simulink model "Torque_Control"  (R2022a)
settings: Solver=FixedStepAuto  StartTime=0.0  StopTime=10.0  RelTol=1e-3
libraries: simulink x9, eeGeneralControl x3
(part 2 of 6)

== system Torque_Control/Power Limitation Temperature/temperature_SoP/temperature_rise_limitator_Motors ==
  note: initial_limitation es una constante para la reducción inicial (de 0 a 1, más bajo significa que cambia
      | menos, más alto la limitación
      | inicial es más bestia).
  note: saturamos de 1 a 0 por si acaso
  note: magia chunga para
      | que los números cuadren
  note: Se limita la corriente en proporción
      | al ratio entre la temperatura actual y 110ºC
  note: output 0 si está por
      | debajo de 110ºC, 1 si está
      | por encima
  max_motor_temp : Inport
  initial_limitation : Inport  Port=2
  Add1 : Sum  Inputs=-+
  Add2 : Sum  Inputs=-++
  Add3 : Sum  Inputs=+-
  Constant1 : Constant  Value=105
  Constant2 : Constant  Value=5
  Constant3 : Constant
  Divide : Product  Inputs=*/
  Low-Pass Filter (Discrete or Continuous) : eeGeneralControl/Low-Pass Filter (Discrete or Continuous)  K=1  T=100  B=inf  A=-inf  init_option=Inherited from block input  x0=0  Ts=-1
  Product4 : Product
  Saturation1 : Saturate  UpperLimit=1  LowerLimit=0
  Temp higher than 110 : simulink/Logic and Bit Operations/Compare To Constant  relop=>=  const=110  OutDataTypeStr=boolean  ZeroCross=off
  SoP : Outport
  wires:
  Divide/1 -> Add3/1
  Constant3/1 -> Add2/3
  Constant1/1 -> Divide/1
  max_motor_temp/1 -> Add1/2, Temp higher than 110/1
  Temp higher than 110/1 -> Add2/1, Product4/2
  Constant2/1 -> Add1/1
  Product4/1 -> Add2/2
  Add2/1 -> Low-Pass Filter (Discrete or Continuous)/1
  Add3/1 -> Product4/1
  Add1/1 -> Divide/2
  Saturation1/1 -> SoP/1
  initial_limitation/1 -> Add3/2
  Low-Pass Filter (Discrete or Continuous)/1 -> Saturation1/1

== system Torque_Control/SAFETY BLOCK/APPS_IMPLAUSIBILITY/Imp ==
  Action Port : ActionPort  ActionPortLabel=if { }
  Constant : Constant  Value=0  OutDataTypeStr=boolean
  Out1 : Outport  VectorParamsAs1DForOutWhenUnconnected=off
  wires:
  Constant/1 -> Out1/1  "Boolean"

== system Torque_Control/SAFETY BLOCK/APPS_IMPLAUSIBILITY/Not Imp ==
  Action Port : ActionPort  ActionPortLabel=else { }
  Constant : Constant  OutDataTypeStr=boolean
  Out1 : Outport  VectorParamsAs1DForOutWhenUnconnected=off
  wires:
  Constant/1 -> Out1/1  "Boolean"

== system Torque_Control/VDC/Regeneration_Enable/Enabled  ==
  In1 : Inport
  Action Port : ActionPort  ActionPortLabel=if { }
  Out1 : Outport  VectorParamsAs1DForOutWhenUnconnected=off
  wires:
  In1/1 -> Out1/1

== system Torque_Control/VDC/Regeneration_Enable/NotEnabled ==
  In1 : Inport
  Action Port : ActionPort  ActionPortLabel=else { }
  Out1 : Outport  VectorParamsAs1DForOutWhenUnconnected=off
  wires:
  In1/1 -> Out1/1

== system Torque_Control/VDC/TEST_MODE_IN/BYPASS ==
  In1 : Inport
  In2 : Inport  Port=2
  In3 : Inport  Port=3
  In4 : Inport  Port=4
  Action Port : ActionPort  ActionPortLabel=else { }
  Out1 : Outport  VectorParamsAs1DForOutWhenUnconnected=off
  Out2 : Outport  Port=2  VectorParamsAs1DForOutWhenUnconnected=off
  Out3 : Outport  Port=3  VectorParamsAs1DForOutWhenUnconnected=off
  Out4 : Outport  Port=4  VectorParamsAs1DForOutWhenUnconnected=off
  wires:
  In1/1 -> Out1/1
  In2/1 -> Out2/1
  In3/1 -> Out3/1
  In4/1 -> Out4/1

== system Torque_Control/VDC/TEST_MODE_IN/TEST_CONSTANTS ==
  Action Port : ActionPort  ActionPortLabel=if { }
  Constant{,1..3} (4 alike) : Constant  Value=800
  Out1 : Outport  VectorParamsAs1DForOutWhenUnconnected=off
  Out2 : Outport  Port=2  VectorParamsAs1DForOutWhenUnconnected=off
  Out3 : Outport  Port=3  VectorParamsAs1DForOutWhenUnconnected=off
  Out4 : Outport  Port=4  VectorParamsAs1DForOutWhenUnconnected=off
  wires:
  Constant/1 -> Out1/1
  Constant1/1 -> Out2/1
  Constant2/1 -> Out3/1
  Constant3/1 -> Out4/1

== system Torque_Control/VDC/Vehicle Dynamics Control Modes/Automatic Failure Mode ==
  In1 : Inport
  Action Port : ActionPort  ActionPortLabel=if { }
  Out1 : Outport  VectorParamsAs1DForOutWhenUnconnected=off
  wires:
  In1/1 -> Out1/1

== system Torque_Control/VDC/Vehicle Dynamics Control Modes/Manual Failure Mode Selection ==
  In1 : Inport
  Action Port : ActionPort  ActionPortLabel=else { }
  Out1 : Outport  VectorParamsAs1DForOutWhenUnconnected=off
  wires:
  In1/1 -> Out1/1

== system Torque_Control/VDC/Vehicle Dynamics Control Modes/Rigid Axle ==
  "Ap_Sat_up " : Inport
  Ap_Sat_down : Inport  Port=2
  Gas Pedal [0-1] : Inport  Port=3
  Max_Motor_Torque_Rear_FM4 [Nm] : Inport  Port=4
  Gear_Ratio_MtoW : Inport  Port=5
  Action Port : ActionPort  ActionPortLabel=elseif { }
  "Rigid Axle without TC " : MATLAB Function  TreatAsAtomicUnit=on
  Tq_RR_FM4 [Nm] (0,inf) : Outport  VectorParamsAs1DForOutWhenUnconnected=off
  Tq_RL_FM4 [Nm] (0,inf) : Outport  Port=2  VectorParamsAs1DForOutWhenUnconnected=off
  wires:
  Max_Motor_Torque_Rear_FM4 [Nm]/1 -> "Rigid Axle without TC "/4(Maximum_Torque_Rear)
  "Rigid Axle without TC "/2(Torque_RL) -> Tq_RL_FM4 [Nm] (0,inf)/1
  "Rigid Axle without TC "/1(Torque_RR) -> Tq_RR_FM4 [Nm] (0,inf)/1
  Gas Pedal [0-1]/1 -> "Rigid Axle without TC "/1(Ap)
  "Ap_Sat_up "/1 -> "Rigid Axle without TC "/2(Ap_Sat_up)
  Ap_Sat_down/1 -> "Rigid Axle without TC "/3(Ap_Sat_down)
  Gear_Ratio_MtoW/1 -> "Rigid Axle without TC "/5(Transmission_Gear_Ratio)

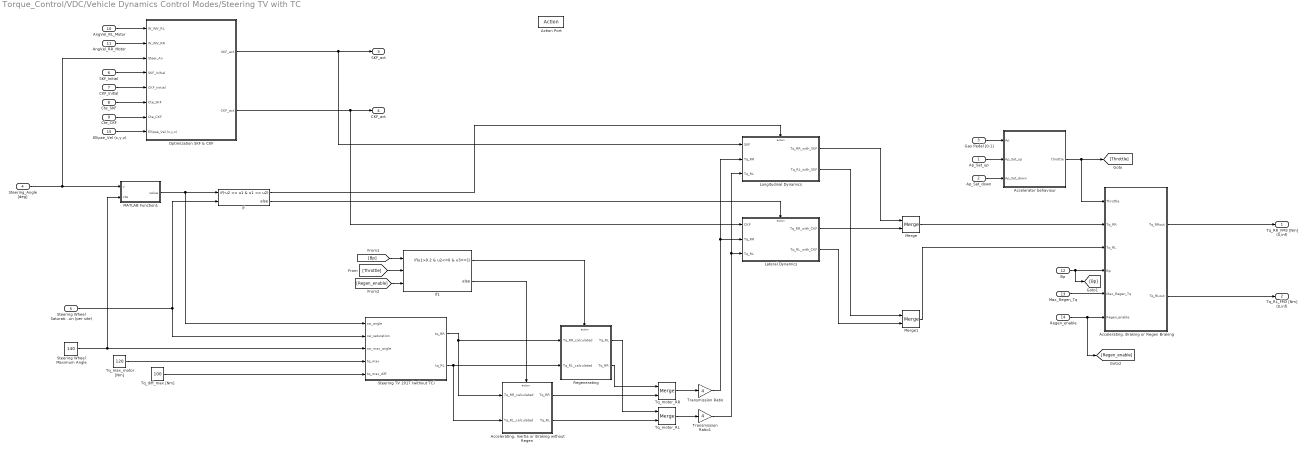
== system Torque_Control/VDC/Vehicle Dynamics Control Modes/Steering TV with TC ==
  "Ap_Sat_up " : Inport
  Ap_Sat_down : Inport  Port=2
  Gas Pedal [0-1] : Inport  Port=3
  Steering_Angle [deg] : Inport  Port=4
  "Steering Wheel Saturation (per site) " : Inport  Port=5
  SKF_Initial : Inport  Port=6
  CKF_Initial : Inport  Port=7
  Cte_SKF : Inport  Port=8
  Cte_CKF : Inport  Port=9
  AngVel_RL_Motor : Inport  Port=10
  AngVel_RR_Motor : Inport  Port=11
  Bp : Inport  Port=12
  Max_Regen_Tq : Inport  Port=13
  Regen_enable : Inport  Port=14
  Ellipse_Vel (x,y,z) : Inport  Port=15
  Action Port : ActionPort  ActionPortLabel=elseif { }
  "Accelerating, Braking or Regen Braking" : Subsystem
  "Accelerating, Inertia or Braking without Regen" : Subsystem  TreatAsAtomicUnit=on
  Accelerator behaviour : MATLAB Function  TreatAsAtomicUnit=on
  If : If  NumInputs=2  IfExpression=-u2 <= u1 & u1 <= u2
  If1 : If  NumInputs=3  IfExpression=u1>0.2 & u2<=0 & u3==1
  Lateral Dynamics : Subsystem  TreatAsAtomicUnit=on
  Longitudinal Dynamics : Subsystem  TreatAsAtomicUnit=on
  MATLAB Function1 : MATLAB Function  TreatAsAtomicUnit=on
  Merge : Merge
  Merge1 : Merge
  Optimization SKF & CKF : Subsystem
  Regenerating : Subsystem  TreatAsAtomicUnit=on
  Steering TV 2017 (without TC) : MATLAB Function  TreatAsAtomicUnit=on
  Steering Wheel Maximum Angle : Constant  Value=140
  Tq_diff_max [Nm] : Constant  Value=100
  Tq_max_motor [Nm] : Constant  Value=120
  Tq_motor_RL : Merge
  Tq_motor_RR : Merge
  Transmission Ratio : Gain  Gain=4
  Transmission Ratio1 : Gain  Gain=4
  Tq_RR_FM3 [Nm] (0,inf) : Outport  VectorParamsAs1DForOutWhenUnconnected=off
  Tq_RL_FM3 [Nm] (0,inf) : Outport  Port=2  VectorParamsAs1DForOutWhenUnconnected=off
  SKF_act : Outport  Port=3  VectorParamsAs1DForOutWhenUnconnected=off
  CKF_act : Outport  Port=4  VectorParamsAs1DForOutWhenUnconnected=off
  wires:
  Steering Wheel Maximum Angle/1 -> Steering TV 2017 (without TC)/3(sw_max_angle), MATLAB Function1/2(cte)
  "Steering Wheel Saturation (per site) "/1 -> Steering TV 2017 (without TC)/2(sw_saturation), If/2
  Transmission Ratio/1 -> Longitudinal Dynamics/2(Tq_RR), Lateral Dynamics/2(Tq_RR)
  Tq_motor_RL/1 -> Transmission Ratio1/1
  MATLAB Function1/1(value) -> Steering TV 2017 (without TC)/1(sw_angle), If/1
  Optimization SKF & CKF/2(CKF_act) -> Lateral Dynamics/1(CKF), CKF_act/1
  SKF_Initial/1 -> Optimization SKF & CKF/4(SKF_Initial)
  Cte_SKF/1 -> Optimization SKF & CKF/6(Cte_SKF)
  AngVel_RL_Motor/1 -> Optimization SKF & CKF/1(W_INV_RL)
  AngVel_RR_Motor/1 -> Optimization SKF & CKF/2(W_INV_RR)
  Optimization SKF & CKF/1(SKF_act) -> Longitudinal Dynamics/1(SKF), SKF_act/1
  Steering_Angle [deg]/1 -> MATLAB Function1/1(v), Optimization SKF & CKF/3(Steer_An)
  CKF_Initial/1 -> Optimization SKF & CKF/5(CKF_Initial)
  Cte_CKF/1 -> Optimization SKF & CKF/7(Cte_CKF)
  If/1 -> Longitudinal Dynamics/Action
  Lateral Dynamics/2(Tq_RL_with_CKF) -> Merge1/2
  If/2 -> Lateral Dynamics/Action
  Longitudinal Dynamics/2(Tq_RL_with_SKF) -> Merge1/1
  Longitudinal Dynamics/1(Tq_RR_with_SKF) -> Merge/1
  Lateral Dynamics/1(Tq_RR_with_CKF) -> Merge/2
  Merge/1 -> "Accelerating, Braking or Regen Braking"/2(Tq_RR)
  Merge1/1 -> "Accelerating, Braking or Regen Braking"/3("Tq_RL ")
  "Accelerating, Braking or Regen Braking"/1(Tq_RRout) -> Tq_RR_FM3 [Nm] (0,inf)/1
  "Accelerating, Braking or Regen Braking"/2(Tq_RLout) -> Tq_RL_FM3 [Nm] (0,inf)/1
  Bp/1 -> [Bp], "Accelerating, Braking or Regen Braking"/4(Bp)
  Max_Regen_Tq/1 -> "Accelerating, Braking or Regen Braking"/5(Max_Regen_Tq)
  Regen_enable/1 -> [Regen_enable], "Accelerating, Braking or Regen Braking"/6(Regen_enable)
  Gas Pedal [0-1]/1 -> Accelerator behaviour/1(Ap)
  "Ap_Sat_up "/1 -> Accelerator behaviour/2(Ap_Sat_up)
  Ap_Sat_down/1 -> Accelerator behaviour/3(Ap_Sat_down)
  Accelerator behaviour/1(throttle) -> [Throttle], "Accelerating, Braking or Regen Braking"/1(Throttle)
  [Throttle] -> If1/2
  [Bp] -> If1/1
  [Regen_enable] -> If1/3
  If1/1 -> Regenerating/Action
  If1/2 -> "Accelerating, Inertia or Braking without Regen"/Action
  Steering TV 2017 (without TC)/2(tq_RL) -> "Accelerating, Inertia or Braking without Regen"/2(Tq_RL_calculated), Regenerating/2(Tq_RL_calculated)
  Steering TV 2017 (without TC)/1(tq_RR) -> "Accelerating, Inertia or Braking without Regen"/1(Tq_RR_calculated), Regenerating/1(Tq_RR_calculated)
  Regenerating/2(Tq_RR) -> Tq_motor_RR/1
  "Accelerating, Inertia or Braking without Regen"/1(Tq_RR) -> Tq_motor_RR/2
  Regenerating/1(Tq_RL) -> Tq_motor_RL/1
  "Accelerating, Inertia or Braking without Regen"/2(Tq_RL) -> Tq_motor_RL/2
  Tq_max_motor [Nm]/1 -> Steering TV 2017 (without TC)/4(tq_max)
  Tq_diff_max [Nm]/1 -> Steering TV 2017 (without TC)/5(tq_max_diff)
  Tq_motor_RR/1 -> Transmission Ratio/1
  Transmission Ratio1/1 -> Longitudinal Dynamics/3(Tq_RL), Lateral Dynamics/3(Tq_RL)
  Ellipse_Vel (x,y,z)/1 -> Optimization SKF & CKF/8(Ellipse_Vel (x,y,z))

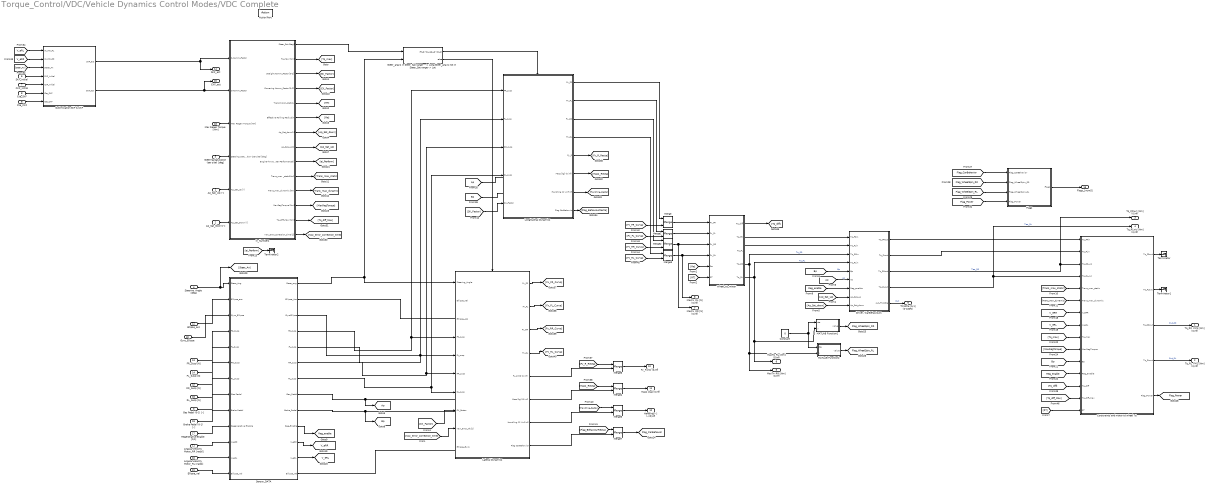
== system Torque_Control/VDC/Vehicle Dynamics Control Modes/VDC Complete ==
  Ap_Sat_Up [-] : Inport
  Ap_Sat_Down [-] : Inport  Port=2
  Gas Pedal (0-1) [-] : Inport  Port=3
  Steering_Angle [deg] : Inport  Port=4
  Steering Saturation (per site) [deg] : Inport  Port=5
  SKF_Initial : Inport  Port=6
  CKF_Initial : Inport  Port=7
  Cte_SKF : Inport  Port=8
  Cte_CKF : Inport  Port=9
  AngularVelocity_Motor_RL [rad/s] : Inport  Port=10
  AngularVelocity_Motor_RR [rad/s] : Inport  Port=11
  Ellipse_acc : Inport  Port=12
  FR_Susp [N] : Inport  Port=13
  FL_Susp [N] : Inport  Port=14
  RR_Susp [N] : Inport  Port=15
  RL_Susp [N] : Inport  Port=16
  Regenerative Enable [0,1] : Inport  Port=17
  Max Regen Torque [Nm] : Inport  Port=18
  Brake Pedal (0-1) [-] : Inport  Port=19
  Gyro_Ellipse : Inport  Port=20
  Ellipse_vel : Inport  Port=21
  Action Port : ActionPort  ActionPortLabel=if { }
  Constant : Constant  Value=0
  Constraints and motor to wheel Tq : Subsystem
  Driver / CarBehaviours : Subsystem
  Flags : Subsystem
  In_Numbers : Subsystem
  Lateral Dynamics : Subsystem  TreatAsAtomicUnit=on
  Longitudinal Dynamics : Subsystem  TreatAsAtomicUnit=on
  MATLAB Function1 : MATLAB Function  TreatAsAtomicUnit=on
  MATLAB Function2 : MATLAB Function  TreatAsAtomicUnit=on
  Merge{,1..7} (8 alike) : Merge
  Optimization SKF & CKF : Subsystem
  Sensor_DATA : Subsystem
  "Steer_ang is in Steer_Sat range ---> Long Steer_ang is not in Steer_Sat range -> Lat " : If  NumInputs=2  IfExpression=u2>=-u1&u2<=u1
  Terminator : Terminator
  Terminator1 : Terminator
  Terminator2 : Terminator
  Wheel_to_motor : Subsystem
  Tq_RR_FM1 [Nm] (0,inf) : Outport  VectorParamsAs1DForOutWhenUnconnected=off
  Tq_RL_FM1 [Nm] (0,inf) : Outport  Port=2  VectorParamsAs1DForOutWhenUnconnected=off
  Tq_RRwc [Nm] (0,inf) : Outport  Port=3  VectorParamsAs1DForOutWhenUnconnected=off
  Tq_RLwc [Nm] (0,inf) : Outport  Port=4  VectorParamsAs1DForOutWhenUnconnected=off
  MaxTq_RR [Nm] (0,inf) : Outport  Port=5  VectorParamsAs1DForOutWhenUnconnected=off
  MaxTq_RL [Nm] (0,inf) : Outport  Port=6  VectorParamsAs1DForOutWhenUnconnected=off
  MaxFx_RR [N] (0,inf) : Outport  Port=7  VectorParamsAs1DForOutWhenUnconnected=off
  MaxFx_RL [N] (0,inf) : Outport  Port=8  VectorParamsAs1DForOutWhenUnconnected=off
  Throttle [0-1] (0-100%) : Outport  Port=9  VectorParamsAs1DForOutWhenUnconnected=off
  Fy_R [N] (0,inf) : Outport  Port=10  VectorParamsAs1DForOutWhenUnconnected=off
  Mass [kg] (0,inf) : Outport  Port=11  VectorParamsAs1DForOutWhenUnconnected=off
  Handling [-] (-inf,inf) : Outport  Port=12  VectorParamsAs1DForOutWhenUnconnected=off
  Flags_[num5] : Outport  Port=13  VectorParamsAs1DForOutWhenUnconnected=off
  SKF_act : Outport  Port=14  VectorParamsAs1DForOutWhenUnconnected=off
  CKF_act : Outport  Port=15  VectorParamsAs1DForOutWhenUnconnected=off
  tag scope: Ap=global, Bp=global, Flag_CarBehavior=global, Flag_Power=global, Flag_WheelSpin_RL=global, Flag_WheelSpin_RR=global, Reg_enable=global, V_eRL=global, V_eRR=global
  wires:
  "Steer_ang is in Steer_Sat range ---> Long Steer_ang is not in Steer_Sat range -> Lat "/1 -> Longitudinal Dynamics/Action
  "Steer_ang is in Steer_Sat range ---> Long Steer_ang is not in Steer_Sat range -> Lat "/2 -> Lateral Dynamics/Action
  Sensor_DATA/7(RL_susp) -> Longitudinal Dynamics/4(RL_susp), Lateral Dynamics/7(RL_susp)
  In_Numbers/3(Straight Kamm_Factor [0-2]) -> [SK_Factor]
  In_Numbers/1(Steer_Sat [deg]) -> "Steer_ang is in Steer_Sat range ---> Long Steer_ang is not in Steer_Sat range -> Lat "/1
  In_Numbers/2(Tq_Max [Nm]) -> [Tq_max]
  Sensor_DATA/8(Gas_Pedal) -> [Ap]
  In_Numbers/6(Effective Rolling Radius[m]) -> [Re]
  In_Numbers/5(Transmision_Ratio[-]) -> [RT]
  Sensor_DATA/6(RR_susp) -> Lateral Dynamics/6(RR_susp), Longitudinal Dynamics/3(RR_susp)
  In_Numbers/8(Ap_Sat_up[-]) -> [Ap_Sat_up]
  In_Numbers/7(Ap_Sat_down[-]) -> [Ap_Sat_down]
  Driver / CarBehaviours/3(Tq_RRout) -> Tq_RRwc [Nm] (0,inf)/1, Constraints and motor to wheel Tq/3(Tq_RR_wc)  "Teo_RR"
  Sensor_DATA/9(Brake_Pedal) -> [Bp]
  Sensor_DATA/5(FL_susp) -> Longitudinal Dynamics/2(FL_susp), Lateral Dynamics/5(FL_susp)
  Sensor_DATA/10(Reg_Enable) -> [Reg_enable]
  Sensor_DATA/4(FR_susp) -> Lateral Dynamics/4(FR_susp), Longitudinal Dynamics/1(FR_susp)
  Sensor_DATA/1(Steer_ang) -> "Steer_ang is in Steer_Sat range ---> Long Steer_ang is not in Steer_Sat range -> Lat "/2, Lateral Dynamics/1(Steering_Angle)
  Wheel_to_motor/5(Tq_RL) -> Driver / CarBehaviours/4("Tq_RLin "), MaxTq_RL [Nm] (0,inf)/1, MATLAB Function1/2(v)  "Tq_RL"
  [Trans_max_dynamic] -> Constraints and motor to wheel Tq/6(Trans_max_dynamic)
  Driver / CarBehaviours/5(out_Throttle) -> Throttle [0-1] (0-100%)/1  "Out"
  Wheel_to_motor/4(Tq_RR) -> Driver / CarBehaviours/3(Tq_RRin), MaxTq_RR [Nm] (0,inf)/1, MATLAB Function2/2(v)  "Tq_RR"
  Wheel_to_motor/3(Tq_FL) -> Driver / CarBehaviours/2(Tq_FLin)
  In_Numbers/11(Trans_max_dynamic [Nm]) -> [Trans_max_dynamic]
  [Reg_enable] -> Driver / CarBehaviours/7(Reg_enable)
  [Ap_Sat_up] -> Driver / CarBehaviours/8(Ap_Sat_up)
  In_Numbers/10(Trans_max _static[Nm]) -> [Trans_max_static]
  [Ap] -> Driver / CarBehaviours/6(Ap)  "Ap"
  [Ap_Sat_down] -> Driver / CarBehaviours/9(Ap_Sat_down)
  Driver / CarBehaviours/4(Tq_RLout) -> Constraints and motor to wheel Tq/4("Tq_RL_wc "), Tq_RLwc [Nm] (0,inf)/1  "Teo_RL"
  Driver / CarBehaviours/2("Tq_FLout ") -> Constraints and motor to wheel Tq/2(Tq_FLin)
  Steering_Angle [deg]/1 -> Sensor_DATA/1(Steer_Ang), [Steer_An]
  Wheel_to_motor/2(Tq_FR) -> Driver / CarBehaviours/1(Tq_FRin)
  Driver / CarBehaviours/1(Tq_FRout) -> Constraints and motor to wheel Tq/1(Tq_FRin)
  [Trans_max_static] -> Constraints and motor to wheel Tq/5("Trans_max_static ")
  [Bp] -> Constraints and motor to wheel Tq/11(Bp)
  Sensor_DATA/12(V_eRL) -> [V_eRL]
  In_Numbers/12(MaxRegTorque [Nm]) -> [MaxRegTorque]
  [Reg_enable] -> Constraints and motor to wheel Tq/12(Reg_enable)
  In_Numbers/9(Engine+Inverter Performance[-]) -> [ei_Perform]
  [Bp] -> Driver / CarBehaviours/5(Bp)  "Bp"
  [Tq_max] -> Constraints and motor to wheel Tq/9(Tq_max)
  RR_Susp [N]/1 -> Sensor_DATA/6(RR_Susp)
  Sensor_DATA/11("V_eRR ") -> [V_eRR]
  [V_eRR] -> Constraints and motor to wheel Tq/7(V_eRR)
  Regenerative Enable [0,1]/1 -> Sensor_DATA/10(Regenerative Enable)
  Brake Pedal (0-1) [-]/1 -> Sensor_DATA/9(Brake Pedal)
  [V_eRL] -> Constraints and motor to wheel Tq/8(V_eRL)
  FL_Susp [N]/1 -> Sensor_DATA/5(FL_Susp)
  FR_Susp [N]/1 -> Sensor_DATA/4(FR_Susp)
  RL_Susp [N]/1 -> Sensor_DATA/7(RL_Susp)
  Gas Pedal (0-1) [-]/1 -> Sensor_DATA/8(Gas Pedal)
  AngularVelocity_Motor_RR [rad/s]/1 -> Sensor_DATA/11(V_eRR)
  AngularVelocity_Motor_RL [rad/s]/1 -> Sensor_DATA/12("V_eRL ")
  Constraints and motor to wheel Tq/1(Tq_FRout) -> Terminator/1
  Constraints and motor to wheel Tq/2("Tq_FLout ") -> Terminator1/1
  In_Numbers/4(Cornering Kamm_Factor [0-2]) -> [CK_Factor]
  [Re] -> Wheel_to_motor/5(Re)
  [RT] -> Wheel_to_motor/6(RT)
  Merge3/1 -> MaxFx_RL [N] (0,inf)/1, Wheel_to_motor/4("Fx_RL ")
  Merge2/1 -> MaxFx_RR [N] (0,inf)/1, Wheel_to_motor/3("Fx_RR ")
  Merge1/1 -> Wheel_to_motor/2("Fx_FL ")
  Max Regen Torque [Nm]/1 -> In_Numbers/3(Max Regen Torque [Nm])
  [CK_Factor] -> Lateral Dynamics/8(CK_Factor)
  [SK_Factor] -> Longitudinal Dynamics/5(SK_Factor)
  Longitudinal Dynamics/1(Fx_FR) -> Merge/1
  Longitudinal Dynamics/2(Fx_FL) -> Merge1/1
  Longitudinal Dynamics/3("Fx_RR ") -> Merge2/1
  Longitudinal Dynamics/4("Fx_RL ") -> Merge3/1
  Merge/1 -> Wheel_to_motor/1("Fx_FR ")
  Steering Saturation (per site) [deg]/1 -> In_Numbers/4(Steering Saturation (per site) [deg])
  Ap_Sat_Up [-]/1 -> In_Numbers/5(Ap_Sat_Up [-])
  Ap_Sat_Down [-]/1 -> In_Numbers/6(Ap_Sat_Down [-])
  [MaxRegTorque] -> Constraints and motor to wheel Tq/10(MaxRegTorque)
  [ei_Perform] -> Terminator2/1
  Merge4/1 -> Mass [kg] (0,inf)/1
  Lateral Dynamics/6(" Mass [kg] (0,inf)") -> Merge4/2
  Lateral Dynamics/7(Handling [-] (-inf,inf)) -> Merge5/2
  Merge5/1 -> Handling [-] (-inf,inf)/1
  Merge6/1 -> Fy_R [N] (0,inf)/1
  Lateral Dynamics/5(Fy_R [N] (0,inf)) -> Merge6/2
  Constraints and motor to wheel Tq/3(Tq_RRout) -> Tq_RR_FM1 [Nm] (0,inf)/1  "Out_RR"
  Constraints and motor to wheel Tq/4(Tq_RLout) -> Tq_RL_FM1 [Nm] (0,inf)/1  "Out_RL"
  Merge7/1 -> [Flag_CarBehavior]
  Lateral Dynamics/8(Flag CarBehavior) -> Merge7/2
  MATLAB Function2/1(value) -> [Flag_WheelSpin_RL]
  MATLAB Function1/1(value) -> [Flag_WheelSpin_RR]
  Constant/1 -> MATLAB Function1/1(cte), MATLAB Function2/1(cte)
  Constraints and motor to wheel Tq/5(Flag_Power) -> [Flag_Power]
  Flags/1(Flags) -> Flags_[num5]/1
  [Flag_WheelSpin_RL] -> Flags/3(Flag_WheelSpin_RL)
  [Flag_WheelSpin_RR] -> Flags/2(Flag_WheelSpin_RR)
  [Flag_CarBehavior] -> Flags/1(Flag_CarBehavior)
  [Flag_Power] -> Flags/4(Flag_Power)
  Optimization SKF & CKF/1(SKF_act) -> In_Numbers/1(S-Kamm_Factor), SKF_act/1
  CKF_Initial/1 -> Optimization SKF & CKF/5(CKF_Initial)
  [Steer_An] -> Optimization SKF & CKF/3(Steer_An)
  [V_eRR] -> Optimization SKF & CKF/2(W_INV_RR)
  Cte_SKF/1 -> Optimization SKF & CKF/6(Cte_SKF)
  Cte_CKF/1 -> Optimization SKF & CKF/7(Cte_CKF)
  SKF_Initial/1 -> Optimization SKF & CKF/4(SKF_Initial)
  [V_eRL] -> Optimization SKF & CKF/1(W_INV_RL)
  Optimization SKF & CKF/2(CKF_act) -> CKF_act/1, In_Numbers/2(C-Kamm_Factor)
  Wheel_to_motor/1(Tq_diff) -> [Tq_diff]
  [Tq_diff] -> Constraints and motor to wheel Tq/13(Tq_diff)
  Ellipse_acc/1 -> Sensor_DATA/2(Ellipse_acc)
  Gyro_Ellipse/1 -> Sensor_DATA/3(Gyro_Ellipse)
  Sensor_DATA/3(GyroEllipse) -> ?
  Sensor_DATA/2(Ellipse_Acc) -> ?
  In_Numbers/14(Yaw_error_correction_time [s]) -> [Yaw_error_correction_time]
  In_Numbers/13(Tq_diff_Max [Nm]) -> [Tq_diff_Max]
  [Yaw_error_correction_time] -> Lateral Dynamics/9(Yaw_error_/dt [s])
  [Ap] -> ?
  [Bp] -> ?
  Longitudinal Dynamics/6(Mass [kg] (0,inf)) -> [Mass_Recta]
  Longitudinal Dynamics/7(Handling [-] (-inf,inf)) -> [Handling_Recta]
  Longitudinal Dynamics/8(Flag CarBehavior) -> [Flag_BehaviourRecta]
  [Fy_R_Recta] -> Merge6/1
  [Mass_Recta] -> Merge4/1
  [Handling_Recta] -> Merge5/1
  [Flag_BehaviourRecta] -> Merge7/1
  Lateral Dynamics/1(Fx_FR) -> [Fx_FR_Curva]
  Lateral Dynamics/2(Fx_FL) -> [Fx_FL_Curva]
  Lateral Dynamics/3("Fx_RR ") -> [Fx_RR_Curva]
  Lateral Dynamics/4("Fx_RL ") -> [Fx_RL_Curva]
  [Fx_FR_Curva] -> Merge/2
  [Fx_FL_Curva] -> Merge1/2
  [Fx_RR_Curva] -> Merge2/2
  [Fx_RL_Curva] -> Merge3/2
  Ellipse_vel/1 -> Sensor_DATA/13(Ellipse_vel)
  Sensor_DATA/13(Ellipse_Vel) -> ?
  [Tq_diff_Max] -> Constraints and motor to wheel Tq/14(Tq_diff_max)
  [RT] -> Constraints and motor to wheel Tq/15(RT)
  Longitudinal Dynamics/5(Fy_R) -> [Fy_R_Recta]

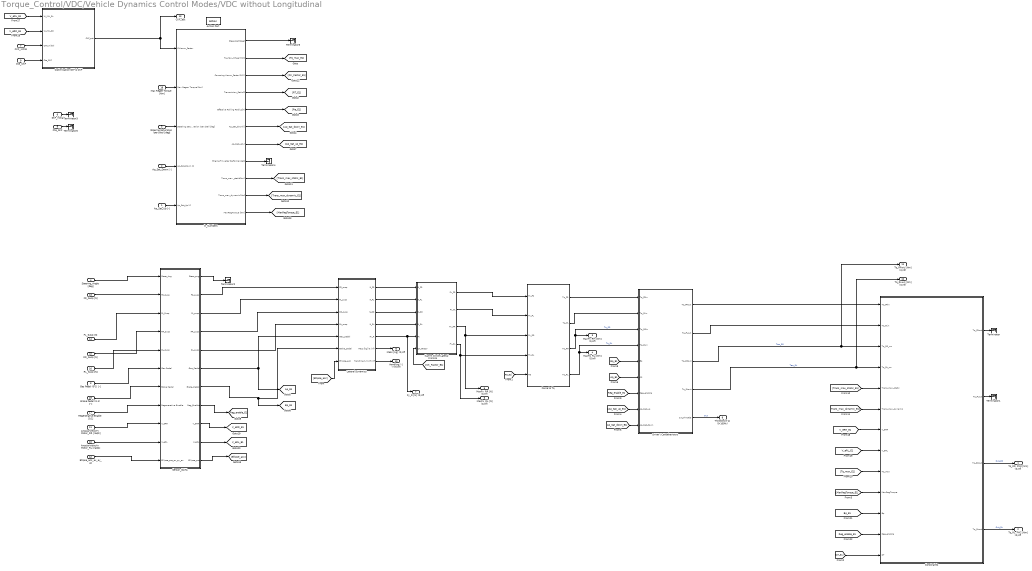
== system Torque_Control/VDC/Vehicle Dynamics Control Modes/VDC without Longitudinal ==
  Ap_Sat_Up [-] : Inport
  Ap_Sat_Down [-] : Inport  Port=2
  Gas Pedal (0-1) [-] : Inport  Port=3
  Steering_Angle [deg] : Inport  Port=4
  Steering Saturation (per site) [deg] : Inport  Port=5
  SKF_initial : Inport  Port=6
  CKF_Initial : Inport  Port=7
  Cte_SKF : Inport  Port=8
  Cte_CKF : Inport  Port=9
  AngularVelocity_Motor_RL [rad/s] : Inport  Port=10
  AngularVelocity_Motor_RR [rad/s] : Inport  Port=11
  Ellipse_acc_ax_ay_az : Inport  Port=12
  FR_Susp [N] : Inport  Port=13
  FL_Susp [N] : Inport  Port=14
  RR_Susp [N] : Inport  Port=15
  RL_Susp [N] : Inport  Port=16
  Regenerative Enable [0,1] : Inport  Port=17
  Max Regen Torque [Nm] : Inport  Port=18
  Brake Pedal (0-1) [-] : Inport  Port=19
  Action Port : ActionPort  ActionPortLabel=elseif { }
  Constraints : Subsystem
  Driver / CarBehaviours : Subsystem
  Force to Tq : Subsystem
  In_Numbers : Subsystem
  Kamm Circle Lateral : Subsystem
  Lateral Dynamics : Subsystem
  Optimization SKF & CKF : Subsystem
  Sensor_DATA : Subsystem
  Terminator{,1..6} (7 alike) : Terminator
  Tq_RR_FM2 [Nm] (0,inf) : Outport  VectorParamsAs1DForOutWhenUnconnected=off
  Tq_RL_FM2 [Nm] (0,inf) : Outport  Port=2  VectorParamsAs1DForOutWhenUnconnected=off
  MaxTq_RR [Nm] (0,inf) : Outport  Port=3  VectorParamsAs1DForOutWhenUnconnected=off
  MaxTq_RL [Nm] (0,inf) : Outport  Port=4  VectorParamsAs1DForOutWhenUnconnected=off
  MaxFx_RR [N] (0,inf) : Outport  Port=5  VectorParamsAs1DForOutWhenUnconnected=off
  MaxFx_RL [N] (0,inf) : Outport  Port=6  VectorParamsAs1DForOutWhenUnconnected=off
  Fy_R [N] (0,inf) : Outport  Port=7  VectorParamsAs1DForOutWhenUnconnected=off
  Throttle [0-1] (0-100%) : Outport  Port=8  VectorParamsAs1DForOutWhenUnconnected=off
  Mass [kg] (0,inf) : Outport  Port=9  VectorParamsAs1DForOutWhenUnconnected=off
  Handling [-] (-inf,inf) : Outport  Port=10  VectorParamsAs1DForOutWhenUnconnected=off
  Tq_RRwc [Nm] (0,inf) : Outport  Port=11  VectorParamsAs1DForOutWhenUnconnected=off
  Tq_RLwc [Nm] (0,inf) : Outport  Port=12  VectorParamsAs1DForOutWhenUnconnected=off
  CKF_act : Outport  Port=13  VectorParamsAs1DForOutWhenUnconnected=off
  tag scope: Ap_E1=global, Bp_E1=global, Reg_enable_E1=global, V_eRL_E1=global, V_eRR_E1=global
  wires:
  Sensor_DATA/5(RL_susp) -> Lateral Dynamics/4(RL_susp)
  In_Numbers/2(Tq_Max_Wheel [Nm]) -> [Tq_max_E1]
  Sensor_DATA/6(Gas_Pedal) -> [Ap_E1], Lateral Dynamics/5(Gas_pedal)
  In_Numbers/5(Effective Rolling Radius[m]) -> [Re_E1]
  In_Numbers/4(Transmision_Ratio[-]) -> [RT_E1]
  Sensor_DATA/4(RR_susp) -> Lateral Dynamics/3(RR_susp)
  In_Numbers/7(Ap_Sat_up[-]) -> [Ap_Sat_up_E1]
  In_Numbers/6(Ap_Sat_down[-]) -> [Ap_Sat_down_E1]
  Sensor_DATA/7(Brake_Pedal) -> Lateral Dynamics/6(Brake_pedal), [Bp_E1]
  Sensor_DATA/3(FL_susp) -> Lateral Dynamics/2(FL_susp)
  Sensor_DATA/8(Reg_Enable) -> [Reg_enable_E1]
  Sensor_DATA/2(FR_susp) -> Lateral Dynamics/1(FR_susp)
  Force to Tq/4(Tq_RL) -> Driver / CarBehaviours/4("Tq_RLin "), MaxTq_RL [Nm] (0,inf)/1  "Tq_RL"
  Force to Tq/3(Tq_RR) -> MaxTq_RR [Nm] (0,inf)/1, Driver / CarBehaviours/3(Tq_RRin)  "Tq_RR"
  In_Numbers/10(Trans_max_dynamic [Nm]) -> [Trans_max_dynamic_E1]
  [Reg_enable_E1] -> Driver / CarBehaviours/7(Reg_enable)
  [Ap_Sat_up_E1] -> Driver / CarBehaviours/8(Ap_Sat_up)
  In_Numbers/9(Trans_max _static[Nm]) -> [Trans_max_static_E1]
  [Ap_E1] -> Driver / CarBehaviours/6(Ap)
  [Ap_Sat_down_E1] -> Driver / CarBehaviours/9(Ap_Sat_down)
  Steering_Angle [deg]/1 -> Sensor_DATA/1(Steer_Ang)
  Sensor_DATA/10(V_eRL) -> [V_eRL_E1]
  In_Numbers/11(MaxRegTorque [Nm]) -> [MaxRegTorque_E1]
  [Bp_E1] -> Driver / CarBehaviours/5(Bp)
  RR_Susp [N]/1 -> Sensor_DATA/4(RR_Susp)
  Sensor_DATA/9("V_eRR ") -> [V_eRR_E1]
  Regenerative Enable [0,1]/1 -> Sensor_DATA/8(Regenerative Enable)
  Brake Pedal (0-1) [-]/1 -> Sensor_DATA/7(Brake Pedal)
  FL_Susp [N]/1 -> Sensor_DATA/3(FL_Susp)
  FR_Susp [N]/1 -> Sensor_DATA/2(FR_Susp)
  RL_Susp [N]/1 -> Sensor_DATA/5(RL_Susp)
  Gas Pedal (0-1) [-]/1 -> Sensor_DATA/6(Gas Pedal)
  AngularVelocity_Motor_RR [rad/s]/1 -> Sensor_DATA/9(V_eRR)
  AngularVelocity_Motor_RL [rad/s]/1 -> Sensor_DATA/10("V_eRL ")
  Max Regen Torque [Nm]/1 -> In_Numbers/2(Max Regen Torque [Nm])
  In_Numbers/3(Cornering Kamm_Factor [0-2]) -> [CK_Factor_E1]
  [Re_E1] -> Force to Tq/5(Re)
  Ap_Sat_Up [-]/1 -> In_Numbers/5(Ap_Sat_Up [-])
  Ap_Sat_Down [-]/1 -> In_Numbers/4(Ap_Sat_Down [-])
  Steering Saturation (per site) [deg]/1 -> In_Numbers/3(Steering Saturation (per site) [deg])
  [CK_Factor_E1] -> Kamm Circle Lateral/6(CK_Factor)
  Kamm Circle Lateral/1(Fx_FR) -> Force to Tq/1("Fx_FR ")
  Kamm Circle Lateral/2(Fx_FL) -> Force to Tq/2("Fx_FL ")
  Kamm Circle Lateral/3("Fx_RR ") -> MaxFx_RR [N] (0,inf)/1, Force to Tq/3("Fx_RR ")
  Kamm Circle Lateral/4("Fx_RL ") -> MaxFx_RL [N] (0,inf)/1, Force to Tq/4("Fx_RL ")
  Sensor_DATA/1(Steer_ang) -> Terminator2/1
  Lateral Dynamics/1(N_FR) -> Kamm Circle Lateral/1("N_FR ")
  Lateral Dynamics/2("N_FL ") -> Kamm Circle Lateral/2(N_FL)
  Lateral Dynamics/3("N_RR ") -> Kamm Circle Lateral/3(N_RR)
  Lateral Dynamics/4(N_RL) -> Kamm Circle Lateral/4(N_RL)
  Driver / CarBehaviours/5(out_Throttle) -> Throttle [0-1] (0-100%)/1  "Out"
  In_Numbers/8(Engine+Inverter Performance[-]) -> Terminator4/1
  In_Numbers/1(Steer_Sat [deg]) -> Terminator5/1
  Lateral Dynamics/6(Mass [kg] (0,inf)) -> Mass [kg] (0,inf)/1
  Lateral Dynamics/7(Handling [-] (-inf,inf)) -> Handling [-] (-inf,inf)/1
  Driver / CarBehaviours/3(Tq_RRout) -> Tq_RRwc [Nm] (0,inf)/1, Constraints/3(Tq_RR_wc)  "Teo_RR"
  [Trans_max_dynamic_E1] -> Constraints/6(Trans_max_dynamic)
  Driver / CarBehaviours/4(Tq_RLout) -> Tq_RLwc [Nm] (0,inf)/1, Constraints/4("Tq_RL_wc ")  "Teo_RL"
  Driver / CarBehaviours/2("Tq_FLout ") -> Constraints/2(Tq_FLin)
  Driver / CarBehaviours/1(Tq_FRout) -> Constraints/1(Tq_FRin)
  [Trans_max_static_E1] -> Constraints/5("Trans_max_static ")
  [Bp_E1] -> Constraints/11(Bp)
  [Reg_enable_E1] -> Constraints/12(Reg_enable)
  [Tq_max_E1] -> Constraints/9(Tq_max)
  [V_eRR_E1] -> Constraints/7(V_eRR)
  [V_eRL_E1] -> Constraints/8(V_eRL)
  Constraints/1(Tq_FRout) -> Terminator/1
  Constraints/2("Tq_FLout ") -> Terminator1/1
  [MaxRegTorque_E1] -> Constraints/10(MaxRegTorque)
  [V_eRR_E1] -> Optimization SKF & CKF/2(W_INV_RR)
  CKF_Initial/1 -> Optimization SKF & CKF/3(CKF_Initial)
  Cte_CKF/1 -> Optimization SKF & CKF/4(Cte_CKF)
  Optimization SKF & CKF/1(CKF_act) -> CKF_act/1, In_Numbers/1(C-Kamm_Factor)
  [V_eRL_E1] -> Optimization SKF & CKF/1(W_INV_RL)
  Ellipse_acc_ax_ay_az/1 -> Sensor_DATA/11(Ellipse_acc_ax_ay_az)
  Sensor_DATA/11(Ellipse_acc) -> [Ellipse_acc]
  Lateral Dynamics/5(Fy_R) -> Kamm Circle Lateral/5(Fy), Fy_R [N] (0,inf)/1
  [Ellipse_acc] -> Lateral Dynamics/7(Ellipse_acc)
  SKF_initial/1 -> Terminator3/1
  Cte_SKF/1 -> Terminator6/1
  Force to Tq/2(Tq_FL) -> Driver / CarBehaviours/2(Tq_FLin)
  Force to Tq/1(Tq_FR) -> Driver / CarBehaviours/1(Tq_FRin)
  [RT_E1] -> Constraints/13(RT)
  Constraints/3(Tq_RRout) -> Tq_RR_FM2 [Nm] (0,inf)/1  "Out_RR"
  Constraints/4(Tq_RLout) -> Tq_RL_FM2 [Nm] (0,inf)/1  "Out_RL"

== system Torque_Control/VDC/WORKSHOP_MODE_RESTRICTIONS/BYPASS ==
  In1 : Inport
  In2 : Inport  Port=2
  Action Port : ActionPort  ActionPortLabel=else { }
  Out1 : Outport  VectorParamsAs1DForOutWhenUnconnected=off
  Out2 : Outport  Port=2  VectorParamsAs1DForOutWhenUnconnected=off
  wires:
  In1/1 -> Out1/1
  In2/1 -> Out2/1

== system Torque_Control/VDC/WORKSHOP_MODE_RESTRICTIONS/Torque_Reduction  ==
  In1 : Inport
  In2 : Inport  Port=2
  Action Port : ActionPort  ActionPortLabel=if { }
  Constant : Constant  Value=15
  Divide : Product  Inputs=*/
  Divide1 : Product  Inputs=*/
  Saturation : Saturate  UpperLimit=10  LowerLimit=-10
  Saturation1 : Saturate  UpperLimit=10  LowerLimit=-10
  Out1 : Outport  VectorParamsAs1DForOutWhenUnconnected=off
  Out2 : Outport  Port=2  VectorParamsAs1DForOutWhenUnconnected=off
  wires:
  Saturation/1 -> Out1/1
  Saturation1/1 -> Out2/1
  In1/1 -> Divide/1
  Divide/1 -> Saturation/1
  In2/1 -> Divide1/1
  Divide1/1 -> Saturation1/1
  Constant/1 -> Divide1/2, Divide/2

== system Torque_Control/Accumulator Power/PowerLimitDetection/OK_OrLatch/Latched Error ==
  Action Port : ActionPort  ActionPortLabel=if { }
  Constant : Constant
  "Out " : Outport  VectorParamsAs1DForOutWhenUnconnected=off
  wires:
  Constant/1 -> "Out "/1

== system Torque_Control/Accumulator Power/PowerLimitDetection/OK_OrLatch/OK ==
  Action Port : ActionPort  ActionPortLabel=else { }
  Constant : Constant  Value=0
  "Out " : Outport  VectorParamsAs1DForOutWhenUnconnected=off
  wires:
  Constant/1 -> "Out "/1

== system Torque_Control/VDC/Vehicle Dynamics Control Modes/Steering TV with TC/Accelerating, Braking or Regen Braking ==
  Throttle : Inport
  Tq_RR : Inport  Port=2
  "Tq_RL " : Inport  Port=3
  Bp : Inport  Port=4
  Max_Regen_Tq : Inport  Port=5
  Regen_enable : Inport  Port=6
  Accelerating : Subsystem  TreatAsAtomicUnit=on
  Braking Conditions : If  NumInputs=3  IfExpression=u1>0.2 & u2<=0 & u3==1  ElseIfExpressions=u1>0.2 & u2<=0 & u3==0, u1<=0.2 & u2<=0
  Inertia Braking : Subsystem  TreatAsAtomicUnit=on
  Mech_Braking : Subsystem  TreatAsAtomicUnit=on
  Merge : Merge  Inputs=4
  Merge1 : Merge  Inputs=4
  Regenerative+Mech Braking : Subsystem  TreatAsAtomicUnit=on
  Tq_RRout : Outport  VectorParamsAs1DForOutWhenUnconnected=off
  Tq_RLout : Outport  Port=2  VectorParamsAs1DForOutWhenUnconnected=off
  wires:
  Braking Conditions/1 -> Regenerative+Mech Braking/Action
  Mech_Braking/2(Tq_RL) -> Merge1/2
  Inertia Braking/1("Tq_RR ") -> Merge/3
  Throttle/1 -> Accelerating/1(Throttle), Braking Conditions/2
  Regenerative+Mech Braking/2(Tq_RL) -> Merge1/1
  Regen_enable/1 -> Braking Conditions/3
  Tq_RR/1 -> Regenerative+Mech Braking/3(RegTq_RR), Accelerating/2(Tq_RR)
  Accelerating/1("Tq_RR ") -> Merge/4
  Regenerative+Mech Braking/1("Tq_RR ") -> Merge/1
  "Tq_RL "/1 -> Regenerative+Mech Braking/4(RegTq_RL), Accelerating/3("Tq_RL ")
  Inertia Braking/2(Tq_RL) -> Merge1/3
  Braking Conditions/4 -> Accelerating/Action
  Braking Conditions/3 -> Inertia Braking/Action
  Bp/1 -> Regenerative+Mech Braking/2(Bp), Braking Conditions/1
  Braking Conditions/2 -> Mech_Braking/Action
  Merge1/1 -> Tq_RLout/1
  Merge/1 -> Tq_RRout/1
  Accelerating/2(Tq_RL) -> Merge1/4
  Mech_Braking/1("Tq_RR ") -> Merge/2
  Max_Regen_Tq/1 -> Regenerative+Mech Braking/1(Max_Regen_Tq)

== system Torque_Control/VDC/Vehicle Dynamics Control Modes/Steering TV with TC/Accelerating, Inertia or Braking without Regen ==
  Tq_RR_calculated : Inport
  Tq_RL_calculated : Inport  Port=2
  Action Port : ActionPort  ActionPortLabel=else { }
  Tq_RR : Outport  VectorParamsAs1DForOutWhenUnconnected=off
  Tq_RL : Outport  Port=2  VectorParamsAs1DForOutWhenUnconnected=off
  wires:
  Tq_RL_calculated/1 -> Tq_RL/1
  Tq_RR_calculated/1 -> Tq_RR/1

== system Torque_Control/VDC/Vehicle Dynamics Control Modes/Steering TV with TC/Lateral Dynamics ==
  CKF : Inport
  Tq_RR : Inport  Port=2
  Tq_RL : Inport  Port=3
  Action Port : ActionPort  ActionPortLabel=else { }
  Product : Product
  Product1 : Product
  Tq_RR_with_CKF : Outport  VectorParamsAs1DForOutWhenUnconnected=off
  Tq_RL_with_CKF : Outport  Port=2  VectorParamsAs1DForOutWhenUnconnected=off
  wires:
  Product1/1 -> Tq_RL_with_CKF/1
  Tq_RR/1 -> Product/1
  Tq_RL/1 -> Product1/1
  CKF/1 -> Product/2, Product1/2
  Product/1 -> Tq_RR_with_CKF/1

== system Torque_Control/VDC/Vehicle Dynamics Control Modes/Steering TV with TC/Longitudinal Dynamics ==
  SKF : Inport
  Tq_RR : Inport  Port=2
  Tq_RL : Inport  Port=3
  Action Port : ActionPort  ActionPortLabel=if { }
  Product : Product
  Product1 : Product
  Tq_RR_with_SKF : Outport  VectorParamsAs1DForOutWhenUnconnected=off
  Tq_RL_with_SKF : Outport  Port=2  VectorParamsAs1DForOutWhenUnconnected=off
  wires:
  Tq_RR/1 -> Product/1
  Tq_RL/1 -> Product1/1
  SKF/1 -> Product/2, Product1/2
  Product/1 -> Tq_RR_with_SKF/1
  Product1/1 -> Tq_RL_with_SKF/1

== system Torque_Control/VDC/Vehicle Dynamics Control Modes/Steering TV with TC/Optimization SKF & CKF ==
  note: Maximum w of both Motors
  W_INV_RL : Inport
  W_INV_RR : Inport  Port=2
  Steer_An : Inport  Port=3
  SKF_Initial : Inport  Port=4
  CKF_Initial : Inport  Port=5
  Cte_SKF : Inport  Port=6
  Cte_CKF : Inport  Port=7
  Ellipse_Vel (x,y,z) : Inport  Port=8
  CKF_prev : DataStoreRead  DataStoreName=B  IndexOptions=Index vector (dialog)  Indices=1  OutputSizes=1
  Constant : Constant  Value=0
  Data Store Memory : DataStoreMemory  ReadBeforeWriteMsg=warning  WriteAfterWriteMsg=warning  WriteAfterReadMsg=warning  ShowAdditionalParam=off
  Data Store Memory1 : DataStoreMemory  DataStoreName=B  ReadBeforeWriteMsg=warning  WriteAfterWriteMsg=warning  WriteAfterReadMsg=warning  ShowAdditionalParam=off
  Data Store Write : DataStoreWrite  IndexOptions=Index vector (dialog)  Indices=1  OutputSizes=1
  Data Store Write1 : DataStoreWrite  DataStoreName=B  IndexOptions=Index vector (dialog)  Indices=1  OutputSizes=1
  Derivative : Derivative
  Display : Display
  Max : MinMax  Function=max  Inputs=2
  Mux : Mux  Inputs=3
  "SKF_prev " : DataStoreRead  IndexOptions=Index vector (dialog)  Indices=1  OutputSizes=1
  Saturation : Saturate  UpperLimit=6000  LowerLimit=0
  Scope : Scope
  Scope1 : Scope
  "Subsystem " : Subsystem
  Switch : Switch  Threshold=900  SaturateOnIntegerOverflow=off  InputSameDT=off
  Terminator : Terminator
  SKF_act : Outport  VectorParamsAs1DForOutWhenUnconnected=off
  CKF_act : Outport  Port=2  VectorParamsAs1DForOutWhenUnconnected=off
  wires:
  SKF_Initial/1 -> "Subsystem "/3(SKF_Initial)
  "Subsystem "/1("SKF_act ") -> SKF_act/1, Data Store Write/1  "SKF"
  Derivative/1 -> "Subsystem "/2(Derivative), Display/1, Switch/1, Switch/2, Saturation/1  "alpha"
  "Subsystem "/2(CKF_act) -> Scope1/1, CKF_act/1, Data Store Write1/1  "CKF"
  Cte_SKF/1 -> "Subsystem "/7(Cte_SKF)
  W_INV_RL/1 -> Mux/1, Max/1  "w (rad/s)"
  Mux/1 -> Scope/1
  Saturation/1 -> Mux/2
  Switch/1 -> Mux/3
  Constant/1 -> Switch/3
  "SKF_prev "/1 -> "Subsystem "/4(SKF_prev)
  CKF_prev/1 -> "Subsystem "/6("CKF_prev ")
  Max/1 -> Derivative/1  "w (rad/s)"
  W_INV_RR/1 -> Max/2
  Cte_CKF/1 -> "Subsystem "/8(Cte_CKF)
  CKF_Initial/1 -> "Subsystem "/5("CKF_Initial ")
  Steer_An/1 -> "Subsystem "/1(Steer_An)
  Ellipse_Vel (x,y,z)/1 -> Terminator/1

== system Torque_Control/VDC/Vehicle Dynamics Control Modes/Steering TV with TC/Regenerating ==
  note: Regenerating: TV inverted because Tq 'negative' when regenerating
  Tq_RR_calculated : Inport
  Tq_RL_calculated : Inport  Port=2
  Action Port : ActionPort  ActionPortLabel=if { }
  Tq_RL : Outport  VectorParamsAs1DForOutWhenUnconnected=off
  Tq_RR : Outport  Port=2  VectorParamsAs1DForOutWhenUnconnected=off
  wires:
  Tq_RR_calculated/1 -> Tq_RL/1
  Tq_RL_calculated/1 -> Tq_RR/1

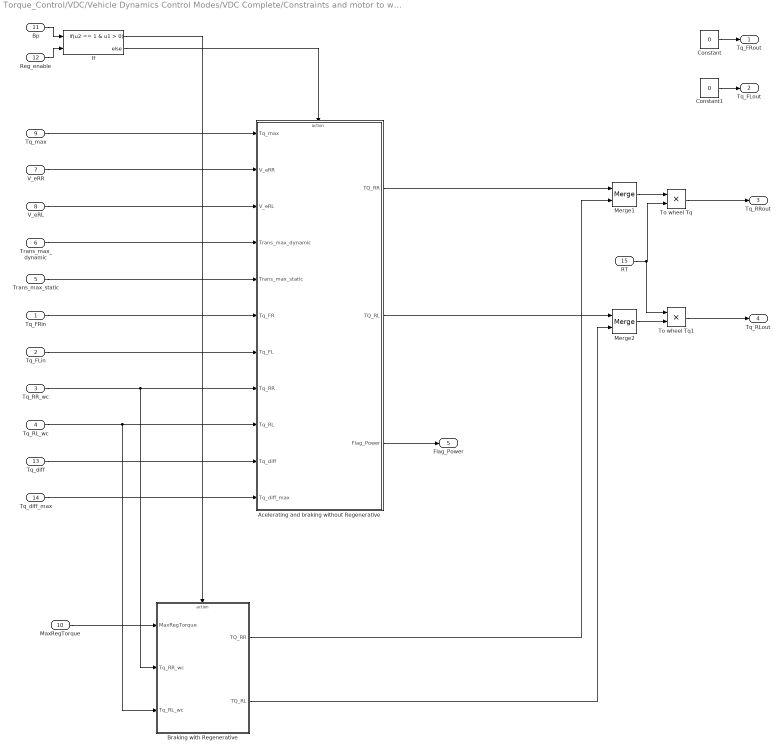
== system Torque_Control/VDC/Vehicle Dynamics Control Modes/VDC Complete/Constraints and motor to wheel Tq ==
  Tq_FRin : Inport
  Tq_FLin : Inport  Port=2
  Tq_RR_wc : Inport  Port=3
  "Tq_RL_wc " : Inport  Port=4
  "Trans_max_static " : Inport  Port=5
  Trans_max_dynamic : Inport  Port=6
  V_eRR : Inport  Port=7
  V_eRL : Inport  Port=8
  Tq_max : Inport  Port=9
  MaxRegTorque : Inport  Port=10
  Bp : Inport  Port=11
  Reg_enable : Inport  Port=12
  Tq_diff : Inport  Port=13
  Tq_diff_max : Inport  Port=14
  RT : Inport  Port=15
  Acelerating and braking without Regenerative : Subsystem  TreatAsAtomicUnit=on
  Braking with Regenerative : Subsystem  TreatAsAtomicUnit=on
  Constant : Constant  Value=0
  Constant1 : Constant  Value=0
  If : If  NumInputs=2  IfExpression=u2 == 1 & u1 > 0
  Merge1 : Merge
  Merge2 : Merge
  To wheel Tq : Product
  To wheel Tq1 : Product
  Tq_FRout : Outport  VectorParamsAs1DForOutWhenUnconnected=off
  "Tq_FLout " : Outport  Port=2  VectorParamsAs1DForOutWhenUnconnected=off
  Tq_RRout : Outport  Port=3  VectorParamsAs1DForOutWhenUnconnected=off
  Tq_RLout : Outport  Port=4  VectorParamsAs1DForOutWhenUnconnected=off
  Flag_Power : Outport  Port=5  VectorParamsAs1DForOutWhenUnconnected=off
  wires:
  Constant1/1 -> "Tq_FLout "/1
  Constant/1 -> Tq_FRout/1
  Tq_RR_wc/1 -> Braking with Regenerative/2(Tq_RR_wc), Acelerating and braking without Regenerative/8(Tq_RR)
  "Tq_RL_wc "/1 -> Braking with Regenerative/3(Tq_RL_wc), Acelerating and braking without Regenerative/9(Tq_RL)
  Tq_max/1 -> Acelerating and braking without Regenerative/1(Tq_max)
  V_eRL/1 -> Acelerating and braking without Regenerative/3(V_eRL)
  Trans_max_dynamic/1 -> Acelerating and braking without Regenerative/4(Trans_max_dynamic)
  "Trans_max_static "/1 -> Acelerating and braking without Regenerative/5(Trans_max_static)
  Merge1/1 -> To wheel Tq/1
  Bp/1 -> If/1
  Reg_enable/1 -> If/2
  V_eRR/1 -> Acelerating and braking without Regenerative/2(V_eRR)
  If/1 -> Braking with Regenerative/Action
  If/2 -> Acelerating and braking without Regenerative/Action
  MaxRegTorque/1 -> Braking with Regenerative/1(MaxRegTorque)
  Tq_FRin/1 -> Acelerating and braking without Regenerative/6(Tq_FR)
  Tq_FLin/1 -> Acelerating and braking without Regenerative/7(Tq_FL)
  Acelerating and braking without Regenerative/2(TQ_RL) -> Merge2/1
  Acelerating and braking without Regenerative/1(TQ_RR) -> Merge1/1
  Braking with Regenerative/1(TQ_RR) -> Merge1/2
  Braking with Regenerative/2(TQ_RL) -> Merge2/2
  Acelerating and braking without Regenerative/3(Flag_Power) -> Flag_Power/1
  Tq_diff/1 -> Acelerating and braking without Regenerative/10(Tq_diff)
  Tq_diff_max/1 -> Acelerating and braking without Regenerative/11(Tq_diff_max)
  RT/1 -> To wheel Tq1/1, To wheel Tq/2
  To wheel Tq/1 -> Tq_RRout/1
  Merge2/1 -> To wheel Tq1/2
  To wheel Tq1/1 -> Tq_RLout/1

== system Torque_Control/VDC/Vehicle Dynamics Control Modes/VDC Complete/Driver // CarBehaviours ==
  Tq_FRin : Inport
  Tq_FLin : Inport  Port=2
  Tq_RRin : Inport  Port=3
  "Tq_RLin " : Inport  Port=4
  Bp : Inport  Port=5
  Ap : Inport  Port=6
  Reg_enable : Inport  Port=7
  Ap_Sat_up : Inport  Port=8
  Ap_Sat_down : Inport  Port=9
  Accelerating : Subsystem  TreatAsAtomicUnit=on
  "Accelerator behaviour " : MATLAB Function  TreatAsAtomicUnit=on
  Braking Conditions : If  NumInputs=3  IfExpression=u1>0.2 & u2<0.1 & u3==1  ElseIfExpressions=u1>0.2 & u2<0.1 & u3==0, u1<0.1 & u2<0.1
  Constant : Constant  Value=0
  Constant1 : Constant  Value=0
  Inertia Braking : Subsystem  TreatAsAtomicUnit=on
  Mech_Braking : Subsystem  TreatAsAtomicUnit=on
  Merge : Merge  Inputs=4
  Merge1 : Merge  Inputs=4
  Regenerative+Mech Braking : Subsystem  TreatAsAtomicUnit=on
  Terminator : Terminator
  Terminator1 : Terminator
  Tq_FRout : Outport  VectorParamsAs1DForOutWhenUnconnected=off
  "Tq_FLout " : Outport  Port=2  VectorParamsAs1DForOutWhenUnconnected=off
  Tq_RRout : Outport  Port=3  VectorParamsAs1DForOutWhenUnconnected=off
  Tq_RLout : Outport  Port=4  VectorParamsAs1DForOutWhenUnconnected=off
  out_Throttle : Outport  Port=5  VectorParamsAs1DForOutWhenUnconnected=off
  wires:
  Constant1/1 -> "Tq_FLout "/1
  Constant/1 -> Tq_FRout/1
  Tq_FLin/1 -> Terminator1/1
  Tq_FRin/1 -> Terminator/1
  Merge/1 -> Tq_RRout/1
  Merge1/1 -> Tq_RLout/1
  Bp/1 -> Regenerative+Mech Braking/1(Bp), Braking Conditions/1
  Regenerative+Mech Braking/1("Tq_RR ") -> Merge/1
  Mech_Braking/1("Tq_RR ") -> Merge/2
  Inertia Braking/1("Tq_RR ") -> Merge/3
  Accelerating/1("Tq_RR ") -> Merge/4
  Regenerative+Mech Braking/2(Tq_RL) -> Merge1/1
  Mech_Braking/2(Tq_RL) -> Merge1/2
  Inertia Braking/2(Tq_RL) -> Merge1/3
  Accelerating/2(Tq_RL) -> Merge1/4
  Braking Conditions/1 -> Regenerative+Mech Braking/Action
  Braking Conditions/2 -> Mech_Braking/Action
  Braking Conditions/3 -> Inertia Braking/Action
  Braking Conditions/4 -> Accelerating/Action
  Tq_RRin/1 -> Accelerating/2(Tq_RR), Regenerative+Mech Braking/2(RegTq_RR)
  "Tq_RLin "/1 -> Accelerating/3("Tq_RL "), Regenerative+Mech Braking/3(RegTq_RL)
  Reg_enable/1 -> Braking Conditions/3
  Accelerating/3(Out_Throttle) -> out_Throttle/1
  "Accelerator behaviour "/1(throttle) -> Accelerating/1(Throttle), Braking Conditions/2
  Ap/1 -> "Accelerator behaviour "/1(Ap)
  Ap_Sat_up/1 -> "Accelerator behaviour "/2(Ap_Sat_up)
  Ap_Sat_down/1 -> "Accelerator behaviour "/3(Ap_Sat_down)

== system Torque_Control/VDC/Vehicle Dynamics Control Modes/VDC Complete/Flags ==
  Flag_CarBehavior : Inport
  Flag_WheelSpin_RR : Inport  Port=2
  Flag_WheelSpin_RL : Inport  Port=3
  Flag_Power : Inport  Port=4
  Mux : Mux
  Flags : Outport  VectorParamsAs1DForOutWhenUnconnected=off
  wires:
  Mux/1 -> Flags/1
  Flag_CarBehavior/1 -> Mux/1
  Flag_WheelSpin_RR/1 -> Mux/2
  Flag_WheelSpin_RL/1 -> Mux/3
  Flag_Power/1 -> Mux/4

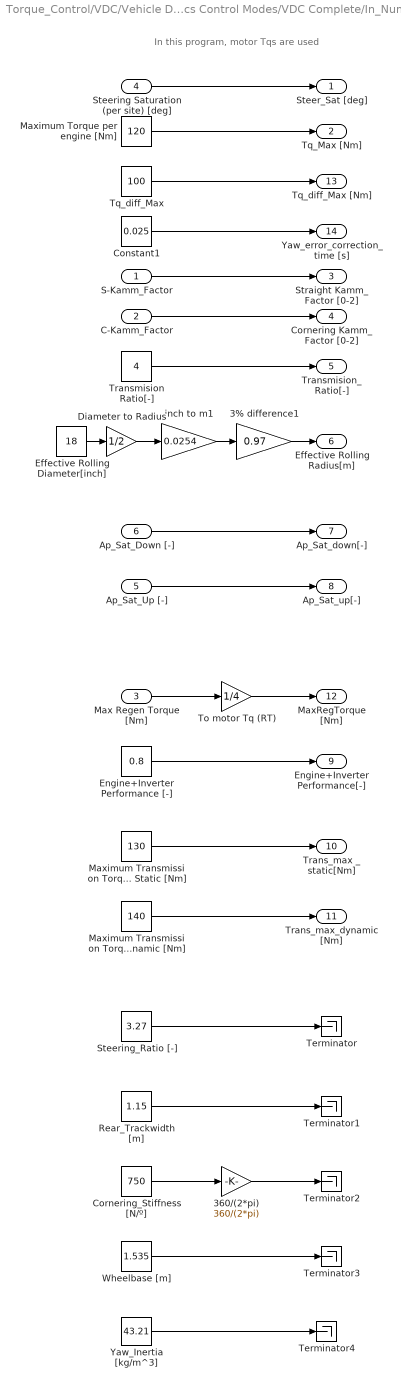
== system Torque_Control/VDC/Vehicle Dynamics Control Modes/VDC Complete/In_Numbers ==
  note: In this program, motor Tqs are used
  S-Kamm_Factor : Inport
  C-Kamm_Factor : Inport  Port=2
  Max Regen Torque [Nm] : Inport  Port=3
  Steering Saturation (per site) [deg] : Inport  Port=4
  Ap_Sat_Up [-] : Inport  Port=5
  Ap_Sat_Down [-] : Inport  Port=6
  3% difference1 : Gain  Gain=0.97
  360/(2*pi) : Gain  Gain=360/(2*pi)
  Constant1 : Constant  Value=0.025
  Cornering_Stiffness [N/º] : Constant  Value=750
  Diameter to Radius : Gain  Gain=1/2
  Effective Rolling Diameter[inch] : Constant  Value=18
  Engine+Inverter Performance [-] : Constant  Value=0.8
  Maximum Torque per engine [Nm] : Constant  Value=120
  Maximum Transmission Torque Dynamic [Nm] : Constant  Value=140
  Maximum Transmission Torque Static [Nm] : Constant  Value=130
  "Rear_Trackwidth [m] " : Constant  Value=1.15
  Steering_Ratio [-] : Constant  Value=3.27
  Terminator{,1..4} (5 alike) : Terminator
  To motor Tq (RT) : Gain  Gain=1/4
  Tq_diff_Max : Constant  Value=100
  Transmision Ratio[-] : Constant  Value=4
  Wheelbase [m] : Constant  Value=1.535
  Yaw_Inertia [kg/m^3] : Constant  Value=43.21  VectorParams1D=off  SampleTime=-1
  inch to m1 : Gain  Gain=0.0254
  Steer_Sat [deg] : Outport  VectorParamsAs1DForOutWhenUnconnected=off
  Tq_Max [Nm] : Outport  Port=2  VectorParamsAs1DForOutWhenUnconnected=off
  Straight Kamm_Factor [0-2] : Outport  Port=3  VectorParamsAs1DForOutWhenUnconnected=off
  Cornering Kamm_Factor [0-2] : Outport  Port=4  VectorParamsAs1DForOutWhenUnconnected=off
  Transmision_Ratio[-] : Outport  Port=5  VectorParamsAs1DForOutWhenUnconnected=off
  Effective Rolling Radius[m] : Outport  Port=6  VectorParamsAs1DForOutWhenUnconnected=off
  Ap_Sat_down[-] : Outport  Port=7  VectorParamsAs1DForOutWhenUnconnected=off
  Ap_Sat_up[-] : Outport  Port=8  VectorParamsAs1DForOutWhenUnconnected=off
  Engine+Inverter Performance[-] : Outport  Port=9  VectorParamsAs1DForOutWhenUnconnected=off
  Trans_max _static[Nm] : Outport  Port=10  VectorParamsAs1DForOutWhenUnconnected=off
  Trans_max_dynamic [Nm] : Outport  Port=11  VectorParamsAs1DForOutWhenUnconnected=off
  MaxRegTorque [Nm] : Outport  Port=12  VectorParamsAs1DForOutWhenUnconnected=off
  Tq_diff_Max [Nm] : Outport  Port=13
  Yaw_error_correction_time [s] : Outport  Port=14
  wires:
  Maximum Torque per engine [Nm]/1 -> Tq_Max [Nm]/1
  Transmision Ratio[-]/1 -> Transmision_Ratio[-]/1
  Maximum Transmission Torque Static [Nm]/1 -> Trans_max _static[Nm]/1
  Maximum Transmission Torque Dynamic [Nm]/1 -> Trans_max_dynamic [Nm]/1
  Engine+Inverter Performance [-]/1 -> Engine+Inverter Performance[-]/1
  S-Kamm_Factor/1 -> Straight Kamm_Factor [0-2]/1
  C-Kamm_Factor/1 -> Cornering Kamm_Factor [0-2]/1
  Steering Saturation (per site) [deg]/1 -> Steer_Sat [deg]/1
  Ap_Sat_Up [-]/1 -> Ap_Sat_up[-]/1
  Ap_Sat_Down [-]/1 -> Ap_Sat_down[-]/1
  Steering_Ratio [-]/1 -> Terminator/1
  "Rear_Trackwidth [m] "/1 -> Terminator1/1
  Cornering_Stiffness [N/º]/1 -> 360/(2*pi)/1
  Wheelbase [m]/1 -> Terminator3/1
  360/(2*pi)/1 -> Terminator2/1
  Yaw_Inertia [kg/m^3]/1 -> Terminator4/1
  Tq_diff_Max/1 -> Tq_diff_Max [Nm]/1
  Constant1/1 -> Yaw_error_correction_time [s]/1
  Effective Rolling Diameter[inch]/1 -> Diameter to Radius/1
  inch to m1/1 -> 3% difference1/1
  Diameter to Radius/1 -> inch to m1/1
  3% difference1/1 -> Effective Rolling Radius[m]/1
  Max Regen Torque [Nm]/1 -> To motor Tq (RT)/1
  To motor Tq (RT)/1 -> MaxRegTorque [Nm]/1

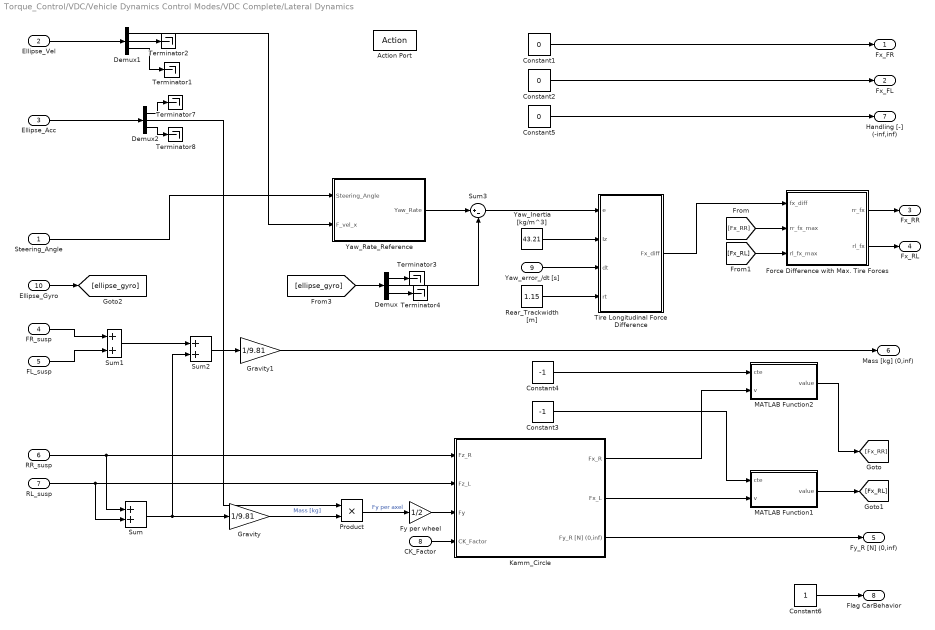
== system Torque_Control/VDC/Vehicle Dynamics Control Modes/VDC Complete/Lateral Dynamics ==
  Steering_Angle : Inport
  Ellipse_Vel : Inport  Port=2
  Ellipse_Acc : Inport  Port=3
  FR_susp : Inport  Port=4
  FL_susp : Inport  Port=5
  RR_susp : Inport  Port=6
  RL_susp : Inport  Port=7
  CK_Factor : Inport  Port=8
  Yaw_error_/dt [s] : Inport  Port=9
  Ellipse_Gyro : Inport  Port=10
  Action Port : ActionPort  ActionPortLabel=else { }
  Constant1 : Constant  Value=0
  Constant2 : Constant  Value=0
  Constant3 : Constant  Value=-1
  Constant4 : Constant  Value=-1
  Constant5 : Constant  Value=0
  Constant6 : Constant
  Demux : Demux  Outputs=3
  Demux1 : Demux  Outputs=3
  Demux2 : Demux  Outputs=3
  Force Difference with Max. Tire Forces : MATLAB Function  TreatAsAtomicUnit=on
  Fy per wheel : Gain  Gain=1/2
  Gravity : Gain  Gain=1/9.81
  Gravity1 : Gain  Gain=1/9.81
  Kamm_Circle : Subsystem
  MATLAB Function1 : MATLAB Function  TreatAsAtomicUnit=on
  MATLAB Function2 : MATLAB Function  TreatAsAtomicUnit=on
  Product : Product
  "Rear_Trackwidth [m] " : Constant  Value=1.15
  Sum : Sum
  Sum1 : Sum
  Sum2 : Sum
  Sum3 : Sum  Inputs=|+-
  Terminator{1..4,7..8} (6 alike) : Terminator
  Tire Longitudinal Force Difference : Subsystem
  Yaw_Inertia [kg/m^3] : Constant  Value=43.21  VectorParams1D=off  SampleTime=-1
  Yaw_Rate_Reference : Subsystem
  Fx_FR : Outport  VectorParamsAs1DForOutWhenUnconnected=off
  Fx_FL : Outport  Port=2  VectorParamsAs1DForOutWhenUnconnected=off
  "Fx_RR " : Outport  Port=3  VectorParamsAs1DForOutWhenUnconnected=off
  "Fx_RL " : Outport  Port=4  VectorParamsAs1DForOutWhenUnconnected=off
  Fy_R [N] (0,inf) : Outport  Port=5  VectorParamsAs1DForOutWhenUnconnected=off
  " Mass [kg] (0,inf)" : Outport  Port=6  VectorParamsAs1DForOutWhenUnconnected=off
  Handling [-] (-inf,inf) : Outport  Port=7  VectorParamsAs1DForOutWhenUnconnected=off
  Flag CarBehavior : Outport  Port=8  VectorParamsAs1DForOutWhenUnconnected=off
  wires:
  Constant6/1 -> Flag CarBehavior/1
  Yaw_error_/dt [s]/1 -> Tire Longitudinal Force Difference/3(dt)
  "Rear_Trackwidth [m] "/1 -> Tire Longitudinal Force Difference/4(rt)
  Yaw_Inertia [kg/m^3]/1 -> Tire Longitudinal Force Difference/2(Iz)
  Tire Longitudinal Force Difference/1(Fx_diff) -> Force Difference with Max. Tire Forces/1(fx_diff)
  Sum3/1 -> Tire Longitudinal Force Difference/1(e)
  Yaw_Rate_Reference/1(Yaw_Rate) -> Sum3/1
  [Fx_RL] -> Force Difference with Max. Tire Forces/3(rl_fx_max)
  [Fx_RR] -> Force Difference with Max. Tire Forces/2(rr_fx_max)
  MATLAB Function1/1(value) -> [Fx_RL]
  MATLAB Function2/1(value) -> [Fx_RR]
  Force Difference with Max. Tire Forces/1(rr_fx) -> "Fx_RR "/1
  Force Difference with Max. Tire Forces/2(rl_fx) -> "Fx_RL "/1
  Steering_Angle/1 -> Yaw_Rate_Reference/1(Steering_Angle)
  Kamm_Circle/1(Fx_R) -> MATLAB Function2/2(v)
  RL_susp/1 -> Kamm_Circle/2(Fz_L), Sum/2
  RR_susp/1 -> Kamm_Circle/1(Fz_R), Sum/1
  FL_susp/1 -> Sum1/2
  FR_susp/1 -> Sum1/1
  Kamm_Circle/2(Fx_L) -> MATLAB Function1/2(v)
  Constant4/1 -> MATLAB Function2/1(cte)
  Constant3/1 -> MATLAB Function1/1(cte)
  Demux1/3 -> Terminator1/1
  Ellipse_Vel/1 -> Demux1/1
  Gravity1/1 -> " Mass [kg] (0,inf)"/1
  Sum2/1 -> Gravity1/1
  Sum1/1 -> Sum2/1
  Gravity/1 -> Product/2  "Mass [kg]"
  Sum/1 -> Gravity/1, Sum2/2
  Kamm_Circle/3(Fy_R [N] (0,inf)) -> Fy_R [N] (0,inf)/1
  CK_Factor/1 -> Kamm_Circle/4(CK_Factor)
  Fy per wheel/1 -> Kamm_Circle/3(Fy)
  Constant2/1 -> Fx_FL/1
  Constant1/1 -> Fx_FR/1
  Product/1 -> Fy per wheel/1  "Fy per axel"
  Demux/2 -> Sum3/2
  Demux2/2 -> Product/1
  Demux2/3 -> Terminator8/1
  Demux2/1 -> Terminator7/1
  Ellipse_Acc/1 -> Demux2/1
  Constant5/1 -> Handling [-] (-inf,inf)/1
  Demux1/2 -> Terminator2/1
  Ellipse_Gyro/1 -> [ellipse_gyro]
  [ellipse_gyro] -> Demux/1
  Demux/1 -> Terminator3/1
  Demux/3 -> Terminator4/1
  Demux1/1 -> Yaw_Rate_Reference/2(F_vel_x)
